simulink model "SecRwLtStFtrstTrgtPosSelc"  (R2018b)
settings: Solver=FixedStepDiscrete  StartTime=0.0  StopTime=10.0  FixedStep=0.01  RelTol=1e-3
undefined symbols (not defined in the file or in its folder): KeSMSw4SAcsMd22SecRwLtStFtrstUpwdDnwdPos_Val, KeSMSw4SAcsMd22SecRwLtStFtrstUpwdDnwdPosMax_Val, KeSMSw4SAcsMd22SecRwLtStFtrstUpwdDnwdPosMin_Val, KeSMSw4SAcsMd26SecRwLtStFtrstUpwdDnwdPos_Val, KeSMSw4SAcsMd26SecRwLtStFtrstUpwdDnwdPosMax_Val, KeSMSw4SAcsMd26SecRwLtStFtrstUpwdDnwdPosMin_Val, KeSMSw4SLegrstCloseMdSecRwLtStFtrstUpwdDnwdPos_Val, KeSMSw4SLegrstCloseMdSecRwLtStFtrstUpwdDnwdPosMax_Val, KeSMSw4SLegrstCloseMdSecRwLtStFtrstUpwdDnwdPosMin_Val, KeSMSw4SLegrstOpenMdSecRwLtStFtrstUpwdDnwdPos_Val, KeSMSw4SLegrstOpenMdSecRwLtStFtrstUpwdDnwdPosMax_Val, KeSMSw4SLegrstOpenMdSecRwLtStFtrstUpwdDnwdPosMin_Val, KeSMSw4sLyingMDSecRwLtStFtrstUpwdDnwdPos_Val, KeSMSw4sLyingMDSecRwLtStFtrstUpwdDnwdPosMax_Val, KeSMSw4sLyingMDSecRwLtStFtrstUpwdDnwdPosMin_Val, KeSMSw4sRecoveryMDSecRwLtStFtrstUpwdDnwdPos_Val, KeSMSw4sRecoveryMDSecRwLtStFtrstUpwdDnwdPosMax_Val, KeSMSw4sRecoveryMDSecRwLtStFtrstUpwdDnwdPosMin_Val, KeSMSw4sVIPMDSecRwLtStFtrstUpwdDnwdPos_Val, KeSMSw4sVIPMDSecRwLtStFtrstUpwdDnwdPosMax_Val, KeSMSw4sVIPMDSecRwLtStFtrstUpwdDnwdPosMin_Val
libraries: TrgtPosSelcLib x8
settings Model: ModifiedHistory=2023.8.1 V2.0.0 CR401790 增加模式21-26  Creator=sn2xws  LastModifiedBy=sn2xws
settings DataIOCC: SaveFormat=StructureWithTime
settings OptimizationCC: DefaultParameterBehavior=Inlined  EnhancedBackFolding=on  PassReuseOutputArgsAs=Individual arguments  ZeroExternalMemoryAtStartup=off  ZeroInternalMemoryAtStartup=off  OptimizeBlockOrder=speed  DifferentSizesBufferReuse=on  OptimizationCustomize=off
settings DebuggingCC: ParameterTunabilityLossMsg=error
settings ModelReferenceCC: ModelReferenceNumInstancesAllowed=Single
settings SFSimCC: MATLABDynamicMemAlloc=off
settings RTWCC: SystemTargetFile=autosar.tlc  GenCodeOnly=on  TemplateMakefile=ert_default_tmf  Description=AUTOSAR  GenerateReport=on  IncludeHyperlinkInReport=on  LaunchReport=on  GenerateTraceInfo=on  GenerateTraceReport=on  GenerateTraceReportSl=on  GenerateTraceReportSf=on  GenerateTraceReportEml=on  GenerateCodeMetricsReport=on
settings CodeAppCC: ForceParamTrailComments=on  IgnoreCustomStorageClasses=off  OperatorAnnotations=on  SimulinkDataObjDesc=on  SFDataObjDesc=on  InsertBlockDesc=on
settings STFCustomTargetCC: TargetLangStandard=C99 (ISO)  MultiwordLength=256  ParMdlRefBuildCompliant=on  CompOptLevelCompliant=on  IncludeMdlTerminateFcn=off  CombineOutputUpdateFcns=on  SuppressErrorStatus=on  ERTCustomFileBanners=on  SupportNonFinite=off  SupportComplex=off  SupportContinuousTime=off  SupportNonInlinedSFcns=off  RemoveResetFunc=on  MATLABClassNameForMDSCustomization=Simulink.SoftwareTarget.ERTCustomization  AutosarCompliant=on  UseToolchainInfoCompliant=on  LookupTableObjectStructAxisOrder=2,1,3,4,...  LUTObjectStructOrderEvenSpacing=Size,Table,Breakpoints  SystemTargetFile=autosar.tlc
settings ERTTargetCC: TargetLangStandard=C99 (ISO)  ConcurrentExecutionCompliant=off  IncludeMdlTerminateFcn=off  SuppressErrorStatus=on  SupportNonFinite=off  SupportComplex=off  ModelStepFunctionPrototypeControlCompliant=off  CPPClassGenCompliant=off  AutosarCompliant=on  LookupTableObjectStructAxisOrder=2,1,3,4,...  LUTObjectStructOrderEvenSpacing=Size,Table,Breakpoints  InlinedParameterPlacement=NonHierarchical  ERTCustomFileTemplate=example_file_process.tlc  ERTFilePackagingFormat=Compact

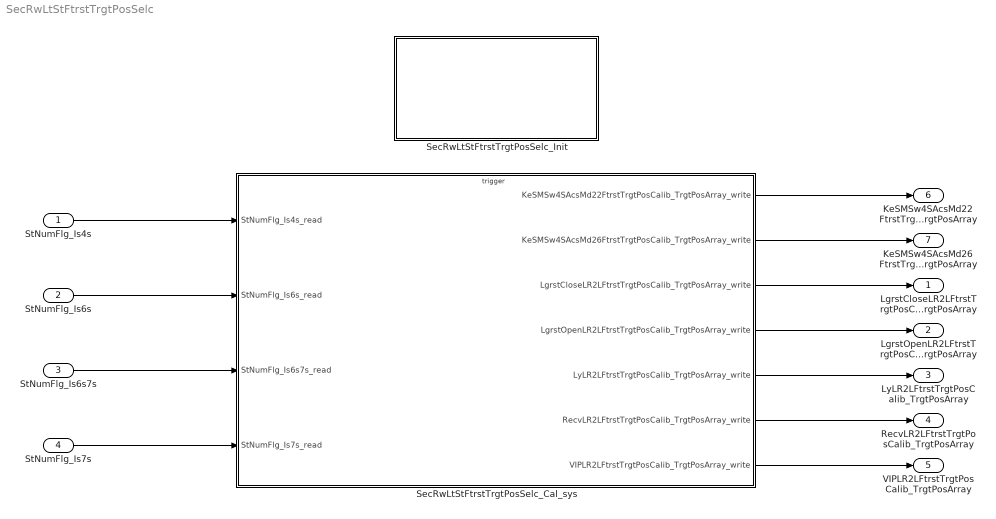
== system SecRwLtStFtrstTrgtPosSelc ==
  StNumFlg_Is4s : Inport  OutDataTypeStr=boolean  PortDimensions=1
  StNumFlg_Is6s : Inport  Port=2  OutDataTypeStr=boolean  PortDimensions=1
  StNumFlg_Is6s7s : Inport  Port=3  OutDataTypeStr=boolean  PortDimensions=1
  StNumFlg_Is7s : Inport  Port=4  OutDataTypeStr=boolean  PortDimensions=1
  SecRwLtStFtrstTrgtPosSelc_Cal_sys : Subsystem
  SecRwLtStFtrstTrgtPosSelc_Init : Subsystem
  LgrstCloseLR2LFtrstTrgtPosCalib_TrgtPosArray : Outport  Description=|  OutDataTypeStr=uint16  PortDimensions=3
      | 0:Pos
      | 1:Max
      | 2:Min
  LgrstOpenLR2LFtrstTrgtPosCalib_TrgtPosArray : Outport  Description=|  Port=2  OutDataTypeStr=uint16  PortDimensions=3
      | 0:Pos
      | 1:Max
      | 2:Min
  LyLR2LFtrstTrgtPosCalib_TrgtPosArray : Outport  Description=|  Port=3  OutDataTypeStr=uint16  PortDimensions=3
      | 0:Pos
      | 1:Max
      | 2:Min
  RecvLR2LFtrstTrgtPosCalib_TrgtPosArray : Outport  Description=|  Port=4  OutDataTypeStr=uint16  PortDimensions=3
      | 0:Pos
      | 1:Max
      | 2:Min
  VIPLR2LFtrstTrgtPosCalib_TrgtPosArray : Outport  Description=|  Port=5  OutDataTypeStr=uint16  PortDimensions=3
      | 0:Pos
      | 1:Max
      | 2:Min
  KeSMSw4SAcsMd22FtrstTrgtPosCalib_TrgtPosArray : Outport  Description=|  Port=6  OutDataTypeStr=uint16  PortDimensions=3
      | 0:Pos
      | 1:Max
      | 2:Min
  KeSMSw4SAcsMd26FtrstTrgtPosCalib_TrgtPosArray : Outport  Description=|  Port=7  OutDataTypeStr=uint16  PortDimensions=3
      | 0:Pos
      | 1:Max
      | 2:Min
  wires:
  StNumFlg_Is4s/1 -> SecRwLtStFtrstTrgtPosSelc_Cal_sys/1(StNumFlg_Is4s_read)
  StNumFlg_Is6s/1 -> SecRwLtStFtrstTrgtPosSelc_Cal_sys/2(StNumFlg_Is6s_read)
  StNumFlg_Is6s7s/1 -> SecRwLtStFtrstTrgtPosSelc_Cal_sys/3(StNumFlg_Is6s7s_read)
  StNumFlg_Is7s/1 -> SecRwLtStFtrstTrgtPosSelc_Cal_sys/4(StNumFlg_Is7s_read)
  SecRwLtStFtrstTrgtPosSelc_Cal_sys/3(LgrstCloseLR2LFtrstTrgtPosCalib_TrgtPosArray_write) -> LgrstCloseLR2LFtrstTrgtPosCalib_TrgtPosArray/1
  SecRwLtStFtrstTrgtPosSelc_Cal_sys/4(LgrstOpenLR2LFtrstTrgtPosCalib_TrgtPosArray_write) -> LgrstOpenLR2LFtrstTrgtPosCalib_TrgtPosArray/1
  SecRwLtStFtrstTrgtPosSelc_Cal_sys/5(LyLR2LFtrstTrgtPosCalib_TrgtPosArray_write) -> LyLR2LFtrstTrgtPosCalib_TrgtPosArray/1
  SecRwLtStFtrstTrgtPosSelc_Cal_sys/6(RecvLR2LFtrstTrgtPosCalib_TrgtPosArray_write) -> RecvLR2LFtrstTrgtPosCalib_TrgtPosArray/1
  SecRwLtStFtrstTrgtPosSelc_Cal_sys/7(VIPLR2LFtrstTrgtPosCalib_TrgtPosArray_write) -> VIPLR2LFtrstTrgtPosCalib_TrgtPosArray/1
  SecRwLtStFtrstTrgtPosSelc_Cal_sys/1(KeSMSw4SAcsMd22FtrstTrgtPosCalib_TrgtPosArray_write) -> KeSMSw4SAcsMd22FtrstTrgtPosCalib_TrgtPosArray/1
  SecRwLtStFtrstTrgtPosSelc_Cal_sys/2(KeSMSw4SAcsMd26FtrstTrgtPosCalib_TrgtPosArray_write) -> KeSMSw4SAcsMd26FtrstTrgtPosCalib_TrgtPosArray/1

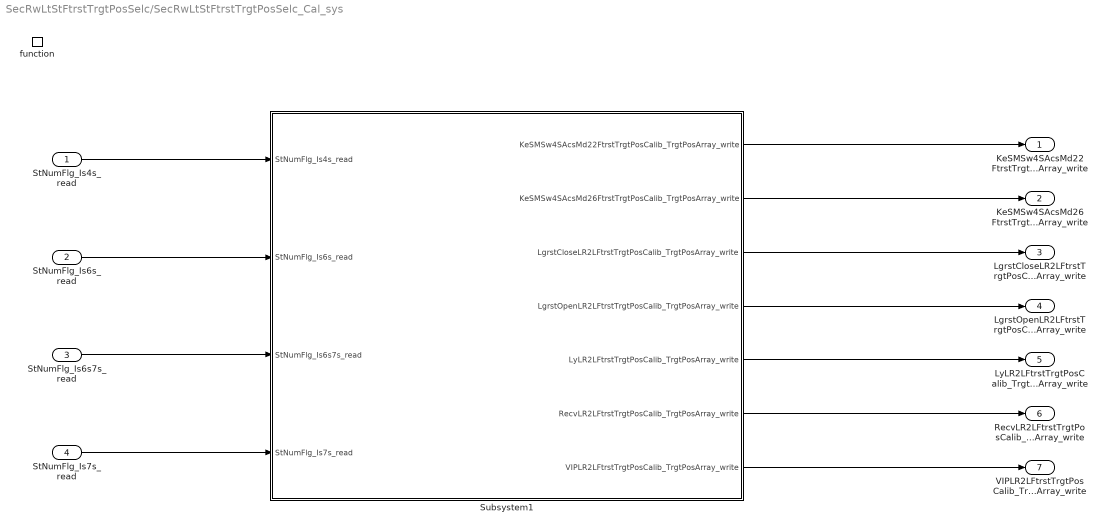
== system SecRwLtStFtrstTrgtPosSelc/SecRwLtStFtrstTrgtPosSelc_Cal_sys ==
  StNumFlg_Is4s_read : Inport
  StNumFlg_Is6s_read : Inport  Port=2
  StNumFlg_Is6s7s_read : Inport  Port=3
  StNumFlg_Is7s_read : Inport  Port=4
  function : TriggerPort  TriggerType=function-call  IsSimulinkFunction=on  FunctionName=SecRwLtStFtrstTrgtPosSelc_Cal  VariantControl=(inherit)
  Subsystem1 : Subsystem
  KeSMSw4SAcsMd22FtrstTrgtPosCalib_TrgtPosArray_write : Outport
      settings: EnsureOutportIsVirtual=on
  KeSMSw4SAcsMd26FtrstTrgtPosCalib_TrgtPosArray_write : Outport  Port=2
      settings: EnsureOutportIsVirtual=on
  LgrstCloseLR2LFtrstTrgtPosCalib_TrgtPosArray_write : Outport  Port=3
      settings: EnsureOutportIsVirtual=on
  LgrstOpenLR2LFtrstTrgtPosCalib_TrgtPosArray_write : Outport  Port=4
      settings: EnsureOutportIsVirtual=on
  LyLR2LFtrstTrgtPosCalib_TrgtPosArray_write : Outport  Port=5
      settings: EnsureOutportIsVirtual=on
  RecvLR2LFtrstTrgtPosCalib_TrgtPosArray_write : Outport  Port=6
      settings: EnsureOutportIsVirtual=on
  VIPLR2LFtrstTrgtPosCalib_TrgtPosArray_write : Outport  Port=7
      settings: EnsureOutportIsVirtual=on
  wires:
  Subsystem1/1(KeSMSw4SAcsMd22FtrstTrgtPosCalib_TrgtPosArray_write) -> KeSMSw4SAcsMd22FtrstTrgtPosCalib_TrgtPosArray_write/1
  Subsystem1/2(KeSMSw4SAcsMd26FtrstTrgtPosCalib_TrgtPosArray_write) -> KeSMSw4SAcsMd26FtrstTrgtPosCalib_TrgtPosArray_write/1
  Subsystem1/3(LgrstCloseLR2LFtrstTrgtPosCalib_TrgtPosArray_write) -> LgrstCloseLR2LFtrstTrgtPosCalib_TrgtPosArray_write/1
  Subsystem1/4(LgrstOpenLR2LFtrstTrgtPosCalib_TrgtPosArray_write) -> LgrstOpenLR2LFtrstTrgtPosCalib_TrgtPosArray_write/1
  Subsystem1/5(LyLR2LFtrstTrgtPosCalib_TrgtPosArray_write) -> LyLR2LFtrstTrgtPosCalib_TrgtPosArray_write/1
  Subsystem1/6(RecvLR2LFtrstTrgtPosCalib_TrgtPosArray_write) -> RecvLR2LFtrstTrgtPosCalib_TrgtPosArray_write/1
  Subsystem1/7(VIPLR2LFtrstTrgtPosCalib_TrgtPosArray_write) -> VIPLR2LFtrstTrgtPosCalib_TrgtPosArray_write/1
  StNumFlg_Is4s_read/1 -> Subsystem1/1(StNumFlg_Is4s_read)
  StNumFlg_Is6s_read/1 -> Subsystem1/2(StNumFlg_Is6s_read)
  StNumFlg_Is6s7s_read/1 -> Subsystem1/3(StNumFlg_Is6s7s_read)
  StNumFlg_Is7s_read/1 -> Subsystem1/4(StNumFlg_Is7s_read)

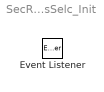
== system SecRwLtStFtrstTrgtPosSelc/SecRwLtStFtrstTrgtPosSelc_Init ==
  Event Listener : EventListener  EventName=reset

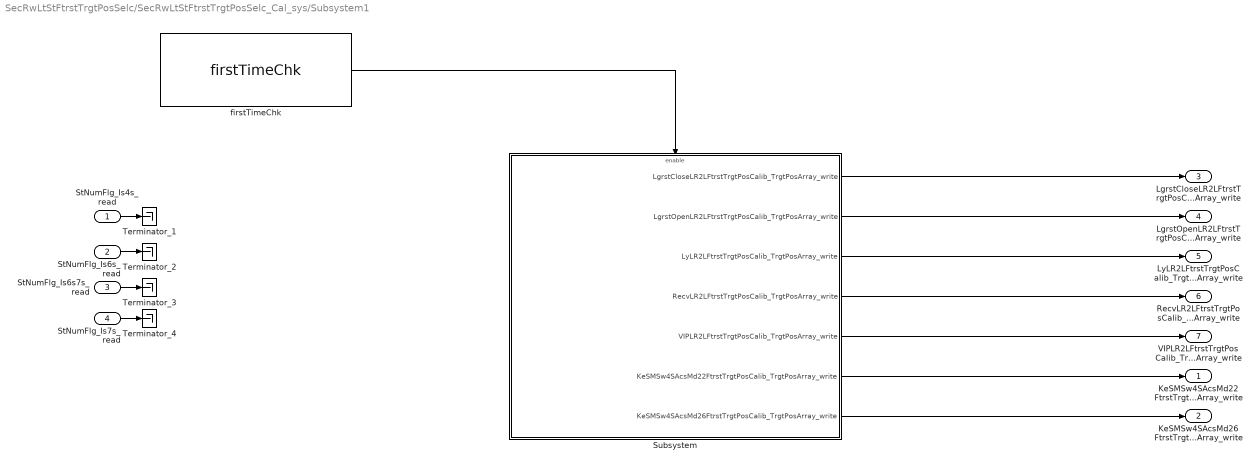
== system SecRwLtStFtrstTrgtPosSelc/SecRwLtStFtrstTrgtPosSelc_Cal_sys/Subsystem1 ==
  StNumFlg_Is4s_read : Inport
  StNumFlg_Is6s_read : Inport  Port=2
  StNumFlg_Is6s7s_read : Inport  Port=3
  StNumFlg_Is7s_read : Inport  Port=4
  Subsystem : Subsystem
  Terminator_{1..4} (4 alike) : Terminator
  firstTimeChk : TrgtPosSelcLib/firstTimeChk  SystemSampleTime=-1
  KeSMSw4SAcsMd22FtrstTrgtPosCalib_TrgtPosArray_write : Outport
      settings: EnsureOutportIsVirtual=on
  KeSMSw4SAcsMd26FtrstTrgtPosCalib_TrgtPosArray_write : Outport  Port=2
      settings: EnsureOutportIsVirtual=on
  LgrstCloseLR2LFtrstTrgtPosCalib_TrgtPosArray_write : Outport  Port=3
      settings: EnsureOutportIsVirtual=on
  LgrstOpenLR2LFtrstTrgtPosCalib_TrgtPosArray_write : Outport  Port=4
      settings: EnsureOutportIsVirtual=on
  LyLR2LFtrstTrgtPosCalib_TrgtPosArray_write : Outport  Port=5
      settings: EnsureOutportIsVirtual=on
  RecvLR2LFtrstTrgtPosCalib_TrgtPosArray_write : Outport  Port=6
      settings: EnsureOutportIsVirtual=on
  VIPLR2LFtrstTrgtPosCalib_TrgtPosArray_write : Outport  Port=7
      settings: EnsureOutportIsVirtual=on
  wires:
  StNumFlg_Is4s_read/1 -> Terminator_1/1
  StNumFlg_Is7s_read/1 -> Terminator_4/1
  Subsystem/3(LyLR2LFtrstTrgtPosCalib_TrgtPosArray_write) -> LyLR2LFtrstTrgtPosCalib_TrgtPosArray_write/1
  StNumFlg_Is6s_read/1 -> Terminator_2/1
  Subsystem/1(LgrstCloseLR2LFtrstTrgtPosCalib_TrgtPosArray_write) -> LgrstCloseLR2LFtrstTrgtPosCalib_TrgtPosArray_write/1
  firstTimeChk/1 -> Subsystem/Enable
  Subsystem/2(LgrstOpenLR2LFtrstTrgtPosCalib_TrgtPosArray_write) -> LgrstOpenLR2LFtrstTrgtPosCalib_TrgtPosArray_write/1
  StNumFlg_Is6s7s_read/1 -> Terminator_3/1
  Subsystem/5(VIPLR2LFtrstTrgtPosCalib_TrgtPosArray_write) -> VIPLR2LFtrstTrgtPosCalib_TrgtPosArray_write/1
  Subsystem/4(RecvLR2LFtrstTrgtPosCalib_TrgtPosArray_write) -> RecvLR2LFtrstTrgtPosCalib_TrgtPosArray_write/1
  Subsystem/7(KeSMSw4SAcsMd26FtrstTrgtPosCalib_TrgtPosArray_write) -> KeSMSw4SAcsMd26FtrstTrgtPosCalib_TrgtPosArray_write/1
  Subsystem/6(KeSMSw4SAcsMd22FtrstTrgtPosCalib_TrgtPosArray_write) -> KeSMSw4SAcsMd22FtrstTrgtPosCalib_TrgtPosArray_write/1

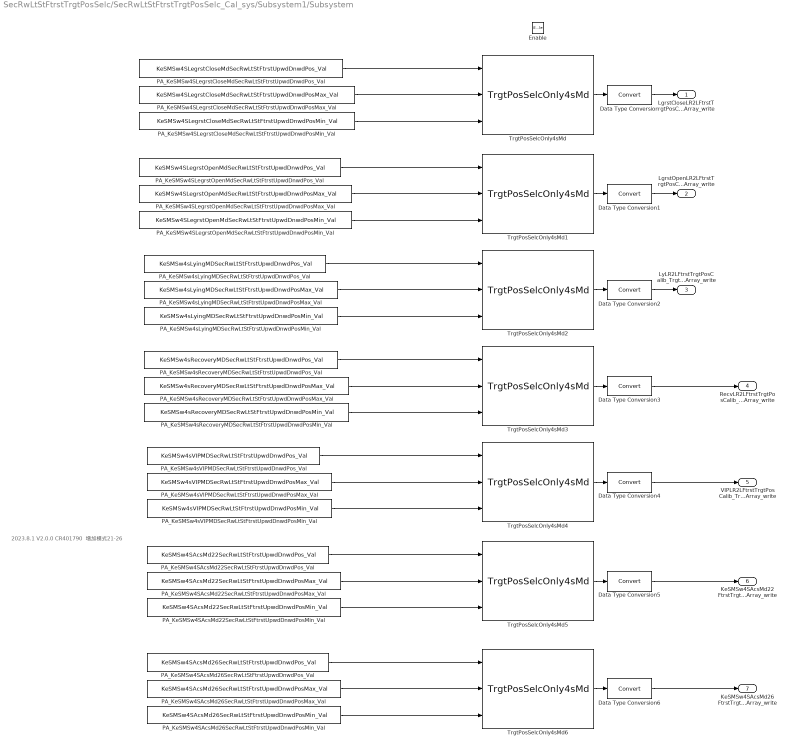
== system SecRwLtStFtrstTrgtPosSelc/SecRwLtStFtrstTrgtPosSelc_Cal_sys/Subsystem1/Subsystem ==
  note: 2023.8.1 V2.0.0 CR401790 增加模式21-26
  Enable : EnablePort
  Data Type Conversion{,1..6} (7 alike) : DataTypeConversion
  PA_KeSMSw4SAcsMd22SecRwLtStFtrstUpwdDnwdPosMax_Val : Constant  Value=KeSMSw4SAcsMd22SecRwLtStFtrstUpwdDnwdPosMax_Val
  PA_KeSMSw4SAcsMd22SecRwLtStFtrstUpwdDnwdPosMin_Val : Constant  Value=KeSMSw4SAcsMd22SecRwLtStFtrstUpwdDnwdPosMin_Val
  PA_KeSMSw4SAcsMd22SecRwLtStFtrstUpwdDnwdPos_Val : Constant  Value=KeSMSw4SAcsMd22SecRwLtStFtrstUpwdDnwdPos_Val
  PA_KeSMSw4SAcsMd26SecRwLtStFtrstUpwdDnwdPosMax_Val : Constant  Value=KeSMSw4SAcsMd26SecRwLtStFtrstUpwdDnwdPosMax_Val
  PA_KeSMSw4SAcsMd26SecRwLtStFtrstUpwdDnwdPosMin_Val : Constant  Value=KeSMSw4SAcsMd26SecRwLtStFtrstUpwdDnwdPosMin_Val
  PA_KeSMSw4SAcsMd26SecRwLtStFtrstUpwdDnwdPos_Val : Constant  Value=KeSMSw4SAcsMd26SecRwLtStFtrstUpwdDnwdPos_Val
  PA_KeSMSw4SLegrstCloseMdSecRwLtStFtrstUpwdDnwdPosMax_Val : Constant  Value=KeSMSw4SLegrstCloseMdSecRwLtStFtrstUpwdDnwdPosMax_Val
  PA_KeSMSw4SLegrstCloseMdSecRwLtStFtrstUpwdDnwdPosMin_Val : Constant  Value=KeSMSw4SLegrstCloseMdSecRwLtStFtrstUpwdDnwdPosMin_Val
  PA_KeSMSw4SLegrstCloseMdSecRwLtStFtrstUpwdDnwdPos_Val : Constant  Value=KeSMSw4SLegrstCloseMdSecRwLtStFtrstUpwdDnwdPos_Val
  PA_KeSMSw4SLegrstOpenMdSecRwLtStFtrstUpwdDnwdPosMax_Val : Constant  Value=KeSMSw4SLegrstOpenMdSecRwLtStFtrstUpwdDnwdPosMax_Val
  PA_KeSMSw4SLegrstOpenMdSecRwLtStFtrstUpwdDnwdPosMin_Val : Constant  Value=KeSMSw4SLegrstOpenMdSecRwLtStFtrstUpwdDnwdPosMin_Val
  PA_KeSMSw4SLegrstOpenMdSecRwLtStFtrstUpwdDnwdPos_Val : Constant  Value=KeSMSw4SLegrstOpenMdSecRwLtStFtrstUpwdDnwdPos_Val
  PA_KeSMSw4sLyingMDSecRwLtStFtrstUpwdDnwdPosMax_Val : Constant  Value=KeSMSw4sLyingMDSecRwLtStFtrstUpwdDnwdPosMax_Val
  PA_KeSMSw4sLyingMDSecRwLtStFtrstUpwdDnwdPosMin_Val : Constant  Value=KeSMSw4sLyingMDSecRwLtStFtrstUpwdDnwdPosMin_Val
  PA_KeSMSw4sLyingMDSecRwLtStFtrstUpwdDnwdPos_Val : Constant  Value=KeSMSw4sLyingMDSecRwLtStFtrstUpwdDnwdPos_Val
  PA_KeSMSw4sRecoveryMDSecRwLtStFtrstUpwdDnwdPosMax_Val : Constant  Value=KeSMSw4sRecoveryMDSecRwLtStFtrstUpwdDnwdPosMax_Val
  PA_KeSMSw4sRecoveryMDSecRwLtStFtrstUpwdDnwdPosMin_Val : Constant  Value=KeSMSw4sRecoveryMDSecRwLtStFtrstUpwdDnwdPosMin_Val
  PA_KeSMSw4sRecoveryMDSecRwLtStFtrstUpwdDnwdPos_Val : Constant  Value=KeSMSw4sRecoveryMDSecRwLtStFtrstUpwdDnwdPos_Val
  PA_KeSMSw4sVIPMDSecRwLtStFtrstUpwdDnwdPosMax_Val : Constant  Value=KeSMSw4sVIPMDSecRwLtStFtrstUpwdDnwdPosMax_Val
  PA_KeSMSw4sVIPMDSecRwLtStFtrstUpwdDnwdPosMin_Val : Constant  Value=KeSMSw4sVIPMDSecRwLtStFtrstUpwdDnwdPosMin_Val
  PA_KeSMSw4sVIPMDSecRwLtStFtrstUpwdDnwdPos_Val : Constant  Value=KeSMSw4sVIPMDSecRwLtStFtrstUpwdDnwdPos_Val
  TrgtPosSelcOnly4sMd{,1..6} (7 alike) : TrgtPosSelcLib/TrgtPosSelcOnly4sMd  SystemSampleTime=-1
  LgrstCloseLR2LFtrstTrgtPosCalib_TrgtPosArray_write : Outport
  LgrstOpenLR2LFtrstTrgtPosCalib_TrgtPosArray_write : Outport  Port=2
  LyLR2LFtrstTrgtPosCalib_TrgtPosArray_write : Outport  Port=3
  RecvLR2LFtrstTrgtPosCalib_TrgtPosArray_write : Outport  Port=4
  VIPLR2LFtrstTrgtPosCalib_TrgtPosArray_write : Outport  Port=5
  KeSMSw4SAcsMd22FtrstTrgtPosCalib_TrgtPosArray_write : Outport  Port=6
  KeSMSw4SAcsMd26FtrstTrgtPosCalib_TrgtPosArray_write : Outport  Port=7
  wires:
  PA_KeSMSw4SLegrstCloseMdSecRwLtStFtrstUpwdDnwdPosMax_Val/1 -> TrgtPosSelcOnly4sMd/2
  PA_KeSMSw4SLegrstCloseMdSecRwLtStFtrstUpwdDnwdPosMin_Val/1 -> TrgtPosSelcOnly4sMd/3
  PA_KeSMSw4sLyingMDSecRwLtStFtrstUpwdDnwdPos_Val/1 -> TrgtPosSelcOnly4sMd2/1
  PA_KeSMSw4SLegrstOpenMdSecRwLtStFtrstUpwdDnwdPos_Val/1 -> TrgtPosSelcOnly4sMd1/1
  PA_KeSMSw4SLegrstOpenMdSecRwLtStFtrstUpwdDnwdPosMax_Val/1 -> TrgtPosSelcOnly4sMd1/2
  PA_KeSMSw4sVIPMDSecRwLtStFtrstUpwdDnwdPosMax_Val/1 -> TrgtPosSelcOnly4sMd4/2
  PA_KeSMSw4sRecoveryMDSecRwLtStFtrstUpwdDnwdPosMin_Val/1 -> TrgtPosSelcOnly4sMd3/3
  PA_KeSMSw4sVIPMDSecRwLtStFtrstUpwdDnwdPosMin_Val/1 -> TrgtPosSelcOnly4sMd4/3
  PA_KeSMSw4SLegrstCloseMdSecRwLtStFtrstUpwdDnwdPos_Val/1 -> TrgtPosSelcOnly4sMd/1
  PA_KeSMSw4sLyingMDSecRwLtStFtrstUpwdDnwdPosMin_Val/1 -> TrgtPosSelcOnly4sMd2/3
  PA_KeSMSw4sVIPMDSecRwLtStFtrstUpwdDnwdPos_Val/1 -> TrgtPosSelcOnly4sMd4/1
  TrgtPosSelcOnly4sMd3/1 -> Data Type Conversion3/1
  PA_KeSMSw4sRecoveryMDSecRwLtStFtrstUpwdDnwdPos_Val/1 -> TrgtPosSelcOnly4sMd3/1
  TrgtPosSelcOnly4sMd/1 -> Data Type Conversion/1
  TrgtPosSelcOnly4sMd1/1 -> Data Type Conversion1/1
  PA_KeSMSw4sLyingMDSecRwLtStFtrstUpwdDnwdPosMax_Val/1 -> TrgtPosSelcOnly4sMd2/2
  PA_KeSMSw4SLegrstOpenMdSecRwLtStFtrstUpwdDnwdPosMin_Val/1 -> TrgtPosSelcOnly4sMd1/3
  PA_KeSMSw4sRecoveryMDSecRwLtStFtrstUpwdDnwdPosMax_Val/1 -> TrgtPosSelcOnly4sMd3/2
  TrgtPosSelcOnly4sMd2/1 -> Data Type Conversion2/1
  TrgtPosSelcOnly4sMd4/1 -> Data Type Conversion4/1
  TrgtPosSelcOnly4sMd5/1 -> Data Type Conversion5/1
  TrgtPosSelcOnly4sMd6/1 -> Data Type Conversion6/1
  PA_KeSMSw4SAcsMd22SecRwLtStFtrstUpwdDnwdPosMax_Val/1 -> TrgtPosSelcOnly4sMd5/2
  PA_KeSMSw4SAcsMd22SecRwLtStFtrstUpwdDnwdPos_Val/1 -> TrgtPosSelcOnly4sMd5/1
  PA_KeSMSw4SAcsMd22SecRwLtStFtrstUpwdDnwdPosMin_Val/1 -> TrgtPosSelcOnly4sMd5/3
  PA_KeSMSw4SAcsMd26SecRwLtStFtrstUpwdDnwdPosMax_Val/1 -> TrgtPosSelcOnly4sMd6/2
  PA_KeSMSw4SAcsMd26SecRwLtStFtrstUpwdDnwdPosMin_Val/1 -> TrgtPosSelcOnly4sMd6/3
  PA_KeSMSw4SAcsMd26SecRwLtStFtrstUpwdDnwdPos_Val/1 -> TrgtPosSelcOnly4sMd6/1
  Data Type Conversion/1 -> LgrstCloseLR2LFtrstTrgtPosCalib_TrgtPosArray_write/1
  Data Type Conversion1/1 -> LgrstOpenLR2LFtrstTrgtPosCalib_TrgtPosArray_write/1
  Data Type Conversion2/1 -> LyLR2LFtrstTrgtPosCalib_TrgtPosArray_write/1
  Data Type Conversion3/1 -> RecvLR2LFtrstTrgtPosCalib_TrgtPosArray_write/1
  Data Type Conversion4/1 -> VIPLR2LFtrstTrgtPosCalib_TrgtPosArray_write/1
  Data Type Conversion5/1 -> KeSMSw4SAcsMd22FtrstTrgtPosCalib_TrgtPosArray_write/1
  Data Type Conversion6/1 -> KeSMSw4SAcsMd26FtrstTrgtPosCalib_TrgtPosArray_write/1
